simulink model "sampleModel1607_sub_sub"  (R2023a)
settings: Solver=VariableStepAuto  StartTime=0.0  StopTime=10.0  RelTol=1e-3
libraries: hdlsllib x2, simulink x1
settings Model: Creator=user1  LastModifiedBy=user1
settings OptimizationCC: BlockReduction=off  ConditionallyExecuteInputs=off

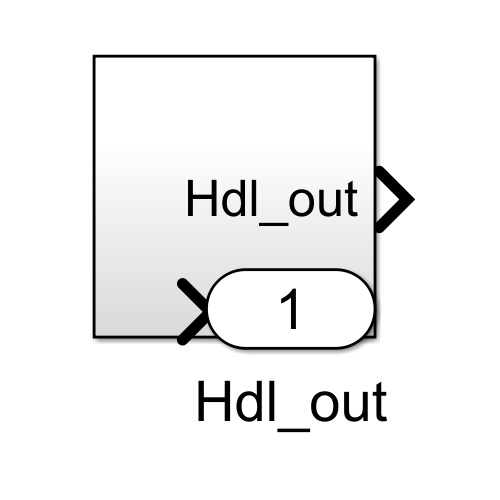
[thumbnail: Simulink's stored preview of the top-level diagram]
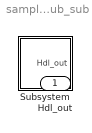
== system sampleModel1607_sub_sub ==
  Subsystem : Subsystem
  Hdl_out : Outport  OutDataTypeStr=uint8

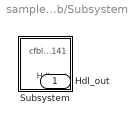
== system sampleModel1607_sub_sub/Subsystem ==
  Subsystem : Subsystem
  Hdl_out : Outport  OutDataTypeStr=uint8

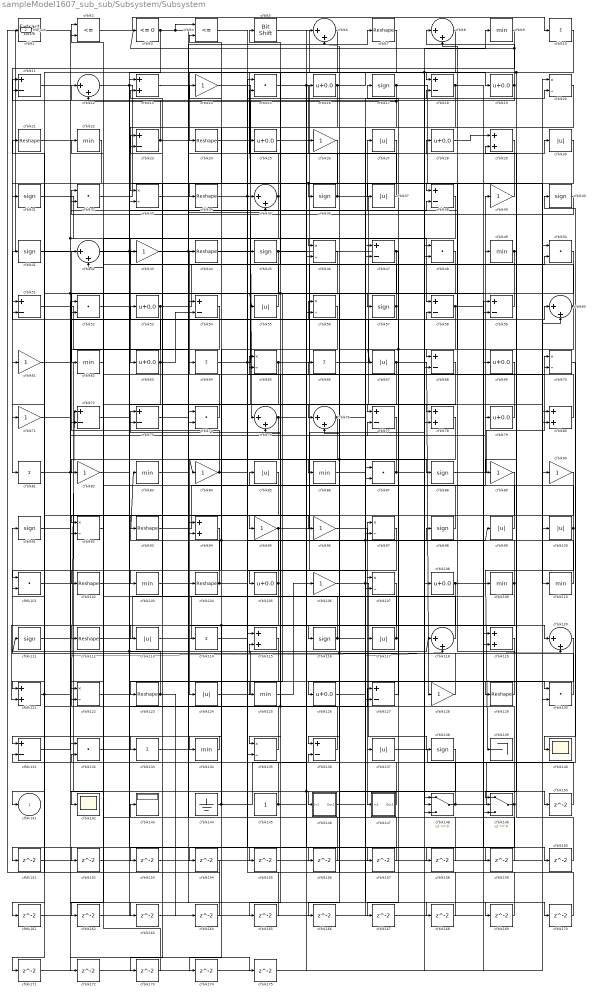
== system sampleModel1607_sub_sub/Subsystem/Subsystem ==
  cfblk1 : simulink/Logic and Bit Operations/Extract Bits  bitsToExtract=Upper half  numBits=8  bitIdxRange=[0 7]  outScalingMode=Preserve fixed-point scaling
      settings: LibrarySourceBlock=|
      | hdlsllib/Logic and Bit
      | Operations/Extract Bits
  cfblk{10,64,66,81,114,133} (6 alike) : Sum  Inputs=+  OutDataTypeStr=uint8
  cfblk{27,30,37,55,67,85,99..100,113,117,124,137} (12 alike) : Abs  OutDataTypeStr=uint8  SaturateOnIntegerOverflow=off
  cfblk{15,32,48,50,52,74,87,101,130,132} (10 alike) : DotProduct  OutDataTypeStr=uint8
  cfblk{7,21,24,34,44,93,102,104,112,123,129} (11 alike) : Reshape
  cfblk{9,22,49,62,83,86,103,109..110,125,134} (11 alike) : MinMax  OutDataTypeStr=uint8
  cfblk{16,19,25,28,53,63,69,79,105,108,126} (11 alike) : Bias  Bias=0.0  SaturateOnIntegerOverflow=off
  cfblk{14,26,39,43,61,71,82,84,89..90,95..96,106,128} (14 alike) : Gain  OutDataTypeStr=uint8
  cfblk{20,33,46,56,65,70,92,97,107,122,135} (11 alike) : Product  Inputs=*/  OutDataTypeStr=uint8  RndMeth=Zero  SaturateOnIntegerOverflow=on
  cfblk{11,18,23,38,47,51,54,58..59,68,72..73,77,127,131,136} (16 alike) : Sum  Inputs=+-  OutDataTypeStr=uint8
  cfblk{17,31,36,40..41,45,57,88,91,98,111,116,138} (13 alike) : Signum
  cfblk{13,29,78,80,94,115,119,121} (8 alike) : Sum  OutDataTypeStr=uint8
  cfblk{6,8,12,35,42,60,75..76,118,120} (10 alike) : Sum  Inputs=|++  OutDataTypeStr=uint8
  cfblk139 : Terminator
  cfblk140 : Scope
  cfblk142 : Scope
  cfblk143 : Display
  cfblk144 : Ground
  cfblk145 : Constant  OutDataTypeStr=uint8  SampleTime=-1
  cfblk146 : Subsystem
      settings: LibrarySourceBlock=|
      | hdlsllib/Ports &
      | Subsystems/Subsystem
  cfblk147 : Subsystem
      settings: LibrarySourceBlock=|
      | hdlsllib/Ports &
      | Subsystems/Subsystem
  cfblk148 : Switch  OutDataTypeStr=uint8  SaturateOnIntegerOverflow=off  InputSameDT=off
  cfblk149 : Switch  OutDataTypeStr=uint8  SaturateOnIntegerOverflow=off  InputSameDT=off
  cfblk{150..175} (26 alike) : Delay  SampleTime=1
  cfblk2 : RelationalOperator  Operator=<=  OutDataTypeStr=boolean  InputSameDT=off
  cfblk3 : hdlsllib/Logic and Bit Operations/Compare To Zero  relop=<=  OutDataTypeStr=uint8
  cfblk4 : RelationalOperator  Operator=<=  OutDataTypeStr=boolean  InputSameDT=off
  cfblk5 : hdlsllib/Logic and Bit Operations/Bit Shift  mode=Shift Left Logical  N=0
  cfblk141 : Outport  OutDataTypeStr=uint8  VectorParamsAs1DForOutWhenUnconnected=off
  Hdl_out : Outport  Port=2  OutDataTypeStr=uint8
  wires:
  cfblk175/1 -> cfblk148/1
  cfblk101/1 -> cfblk175/1
  cfblk174/1 -> cfblk130/2
  cfblk173/1 -> cfblk72/2
  cfblk172/1 -> cfblk59/1
  cfblk71/1 -> cfblk172/1
  cfblk171/1 -> cfblk56/2
  cfblk170/1 -> cfblk87/1
  cfblk86/1 -> cfblk170/1
  cfblk169/1 -> cfblk136/2
  cfblk168/1 -> cfblk15/1
  cfblk167/1 -> cfblk148/3
  cfblk166/1 -> cfblk47/1
  cfblk138/1 -> cfblk166/1
  cfblk165/1 -> cfblk115/1
  cfblk164/1 -> cfblk131/2
  cfblk163/1 -> cfblk119/2
  cfblk91/1 -> cfblk163/1
  cfblk162/1 -> cfblk33/2
  cfblk161/1 -> cfblk78/2
  cfblk160/1 -> cfblk29/2
  cfblk159/1 -> cfblk76/2
  cfblk158/1 -> cfblk74/1
  cfblk13/1 -> cfblk158/1
  cfblk157/1 -> cfblk122/2
  cfblk156/1 -> cfblk42/2
  cfblk4/1 -> cfblk156/1
  cfblk155/1 -> cfblk80/1
  cfblk77/1 -> cfblk155/1
  cfblk154/1 -> cfblk1/1
  cfblk153/1 -> cfblk50/1
  cfblk54/1 -> cfblk153/1
  cfblk152/1 -> cfblk35/1
  cfblk92/1 -> cfblk152/1
  cfblk151/1 -> cfblk127/2
  cfblk150/1 -> cfblk132/2
  cfblk145/1 -> cfblk60/1, cfblk149/2, cfblk101/2
  cfblk103/1 -> cfblk77/2
  cfblk40/1 -> cfblk32/2
  cfblk43/1 -> cfblk114/1, cfblk28/1
  cfblk29/1 -> cfblk36/1, cfblk161/1
  cfblk133/1 -> cfblk94/1
  cfblk30/1 -> cfblk68/1
  cfblk34/1 -> cfblk88/1, cfblk26/1
  cfblk148/1 -> cfblk90/1, cfblk52/2
  cfblk52/1 -> cfblk80/2
  cfblk146/1(Out1) -> cfblk97/2
  cfblk81/1 -> cfblk53/1, cfblk96/1
  cfblk66/1 -> cfblk58/2
  cfblk115/1 -> cfblk134/1
  cfblk83/1 -> cfblk7/1
  cfblk112/1 -> cfblk69/1
  cfblk124/1 -> cfblk48/2
  cfblk73/1 -> cfblk86/1
  cfblk114/1 -> cfblk70/2
  cfblk11/1 -> cfblk47/2, cfblk168/1
  cfblk23/1 -> cfblk11/1, cfblk169/1
  cfblk95/1 -> cfblk48/1, cfblk141/1
  cfblk70/1 -> cfblk140/1
  cfblk50/1 -> cfblk136/1
  cfblk53/1 -> cfblk20/1, cfblk92/2
  cfblk58/1 -> cfblk76/1, cfblk160/1
  cfblk74/1 -> cfblk12/1
  cfblk85/1 -> cfblk101/1
  cfblk69/1 -> cfblk65/2
  cfblk113/1 -> cfblk45/1
  cfblk118/1 -> cfblk13/2
  cfblk12/1 -> cfblk108/1, cfblk18/1, cfblk154/1
  cfblk1/1 -> cfblk59/2, cfblk120/2
  cfblk122/1 -> cfblk50/2, cfblk118/1
  cfblk87/1 -> cfblk82/1, cfblk9/1
  cfblk51/1 -> cfblk74/2
  cfblk90/1 -> cfblk122/1
  cfblk131/1 -> cfblk52/1
  cfblk45/1 -> cfblk62/1, cfblk159/1
  cfblk147/1(Out1) -> cfblk51/1
  cfblk144/1 -> cfblk64/1, cfblk6/1
  cfblk25/1 -> cfblk58/1
  cfblk33/1 -> cfblk35/2
  cfblk56/1 -> cfblk104/1
  cfblk72/1 -> cfblk78/1
  cfblk46/1 -> cfblk121/1
  cfblk16/1 -> cfblk34/1, cfblk19/1
  cfblk100/1 -> cfblk109/1, cfblk23/2
  cfblk80/1 -> cfblk8/2
  cfblk59/1 -> cfblk57/1
  cfblk102/1 -> cfblk13/1
  cfblk121/1 -> cfblk150/1, cfblk151/1
  cfblk48/1 -> cfblk103/1
  cfblk5/1 -> cfblk148/2
  cfblk63/1 -> cfblk41/1, cfblk92/1, cfblk54/2
  cfblk88/1 -> cfblk70/1
  cfblk19/1 -> cfblk8/1, cfblk3/1, cfblk11/2
  cfblk111/1 -> cfblk79/1
  cfblk18/1 -> cfblk119/1, cfblk87/2
  cfblk116/1 -> cfblk2/2, cfblk149/3
  cfblk89/1 -> cfblk95/1
  cfblk42/1 -> cfblk38/2, cfblk130/1
  cfblk28/1 -> cfblk29/1
  cfblk128/1 -> cfblk111/1, cfblk6/2
  cfblk127/1 -> cfblk97/1
  cfblk76/1 -> cfblk30/1, cfblk94/2
  cfblk79/1 -> cfblk44/1
  cfblk126/1 -> cfblk99/1, cfblk20/2
  cfblk14/1 -> cfblk37/1
  cfblk7/1 -> cfblk75/2
  cfblk38/1 -> cfblk142/1
  cfblk37/1 -> cfblk16/1
  cfblk17/1 -> cfblk33/1, cfblk12/2, cfblk60/2
  cfblk119/1 -> cfblk115/2
  cfblk105/1 -> cfblk14/1, cfblk173/1
  cfblk129/1 -> cfblk32/1
  cfblk134/1 -> cfblk131/1
  cfblk135/1 -> cfblk21/1
  cfblk8/1 -> cfblk24/1
  cfblk94/1 -> cfblk112/1
  cfblk98/1 -> cfblk2/1
  cfblk68/1 -> cfblk135/2
  cfblk20/1 -> cfblk105/1
  cfblk132/1 -> cfblk127/1
  cfblk49/1 -> cfblk117/1, cfblk89/1
  cfblk82/1 -> cfblk56/1
  cfblk104/1 -> cfblk73/2, cfblk98/1
  cfblk109/1 -> cfblk43/1, cfblk162/1
  cfblk57/1 -> cfblk5/1, cfblk51/2
  cfblk130/1 -> cfblk17/1
  cfblk39/1 -> cfblk31/1
  cfblk117/1 -> cfblk4/2, cfblk157/1
  cfblk36/1 -> cfblk110/1, cfblk25/1
  cfblk123/1 -> cfblk91/1, cfblk164/1
  cfblk106/1 -> cfblk138/1, cfblk118/2
  cfblk96/1 -> cfblk137/1
  cfblk22/1 -> cfblk61/1
  cfblk21/1 -> cfblk46/2
  cfblk149/1 -> cfblk66/1, cfblk171/1
  cfblk137/1 -> cfblk40/1
  cfblk55/1 -> cfblk22/1
  cfblk26/1 -> cfblk93/1
  cfblk65/1 -> cfblk49/1, cfblk113/1
  cfblk107/1 -> cfblk133/1, cfblk174/1
  cfblk60/1 -> cfblk126/1, cfblk23/1
  cfblk31/1 -> cfblk46/1
  cfblk62/1 -> cfblk102/1
  cfblk3/1 -> cfblk4/1, cfblk120/1, cfblk71/1
  cfblk99/1 -> cfblk65/1
  cfblk15/1 -> cfblk147/1(In1), cfblk107/2
  cfblk67/1 -> cfblk128/1, cfblk125/1
  cfblk32/1 -> cfblk38/1
  cfblk41/1 -> cfblk132/1
  cfblk97/1 -> cfblk135/1
  cfblk93/1 -> cfblk39/1
  cfblk125/1 -> cfblk106/1
  cfblk24/1 -> cfblk100/1
  cfblk110/1 -> cfblk83/1, cfblk54/1
  cfblk108/1 -> cfblk139/1, cfblk121/2
  cfblk78/1 -> cfblk84/1, cfblk116/1
  cfblk120/1 -> cfblk143/1
  cfblk136/1 -> cfblk72/1, cfblk85/1
  cfblk44/1 -> cfblk77/1
  cfblk2/1 -> cfblk10/1
  cfblk84/1 -> cfblk42/1, cfblk18/2
  cfblk75/1 -> cfblk124/1, cfblk129/1
  cfblk61/1 -> cfblk146/1(In1)
  cfblk6/1 -> cfblk55/1, cfblk165/1
  cfblk35/1 -> cfblk63/1, cfblk15/2
  cfblk64/1 -> cfblk27/1, cfblk107/1
  cfblk47/1 -> cfblk67/1, cfblk167/1, cfblk123/1, Hdl_out/1
  cfblk9/1 -> cfblk81/1
  cfblk27/1 -> cfblk73/1
  cfblk10/1 -> cfblk75/1, cfblk68/2, cfblk149/1

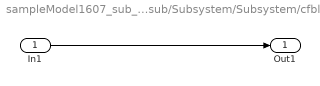
== system sampleModel1607_sub_sub/Subsystem/Subsystem/cfblk146 ==
  In1 : Inport
  Out1 : Outport
  wires:
  In1/1 -> Out1/1

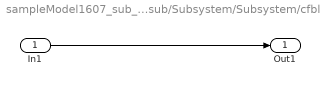
== system sampleModel1607_sub_sub/Subsystem/Subsystem/cfblk147 ==
  In1 : Inport
  Out1 : Outport
  wires:
  In1/1 -> Out1/1
